simulink model "Comparativa_dinamica_ampliado_complejo"  (Simulink 8.3)
settings: Solver=ode45  StartTime=0.0  StopTime=10.0  RelTol=1e-3
settings Model: Creator=mvelasco  LastModifiedBy=mvelasco
settings DataIOCC: SignalLoggingSaveFormat=Dataset
settings DebuggingCC: UnderspecifiedInitializationDetection=Simplified  StateNameClashWarn=none
settings GRTTargetCC: CombineOutputUpdateFcns=on  GRTInterface=off

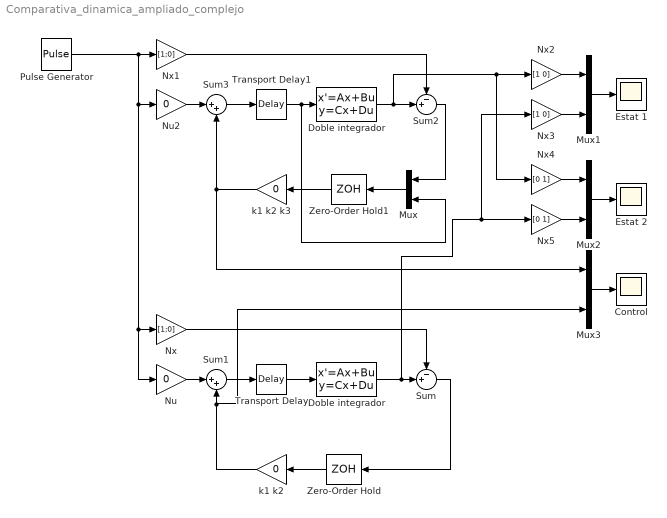
== system Comparativa_dinamica_ampliado_complejo ==
  Control : Scope
      settings: SaveName=ScopeData2
  Doble integrador : StateSpace  X0=0
  "Doble integrador " : StateSpace  X0=0
  Estat 1 : Scope
  Estat 2 : Scope
  Mux{,1..3} (4 alike) : Mux  Inputs=2
  Nu : Gain  Gain=0
  Nu2 : Gain  Gain=0
  Nx : Gain  Gain=[1;0]
  Nx1 : Gain  Gain=[1;0]
  Nx2 : Gain  Gain=[1 0]
  Nx3 : Gain  Gain=[1 0]
  Nx4 : Gain  Gain=[0 1]
  Nx5 : Gain  Gain=[0 1]
  Pulse Generator : DiscretePulseGenerator  PulseType=Time based  Amplitude=3  Period=1  PulseWidth=.5
  Sum : Sum  Inputs=-+|
  Sum1 : Sum  Inputs=|++
  Sum2 : Sum  Inputs=-+|
  Sum3 : Sum  Inputs=|++
  Transport Delay : TransportDelay
  Transport Delay1 : TransportDelay
  Zero-Order Hold : ZeroOrderHold
  Zero-Order Hold1 : ZeroOrderHold
  k1 k2 : Gain  Gain=0
  k1 k2 k3 : Gain  Gain=0
  wires:
  Pulse Generator/1 -> Nu/1, Nx/1, Nu2/1, Nx1/1
  Nx/1 -> Sum/1
  Doble integrador/1 -> Nx3/1, Nx5/1, Sum/2
  Sum/1 -> Zero-Order Hold/1
  k1 k2/1 -> Mux3/2, Sum1/2
  Nu/1 -> Sum1/1
  Sum1/1 -> Transport Delay/1
  Transport Delay/1 -> Doble integrador/1
  Zero-Order Hold/1 -> k1 k2/1
  Nx1/1 -> Sum2/1
  "Doble integrador "/1 -> Nx4/1, Nx2/1, Sum2/2
  k1 k2 k3/1 -> Mux3/1, Sum3/2
  Nu2/1 -> Sum3/1
  Sum3/1 -> Transport Delay1/1
  Transport Delay1/1 -> Mux/2, "Doble integrador "/1
  Zero-Order Hold1/1 -> k1 k2 k3/1
  Mux/1 -> Zero-Order Hold1/1
  Sum2/1 -> Mux/1
  Mux1/1 -> Estat 1/1
  Nx2/1 -> Mux1/1
  Nx3/1 -> Mux1/2
  Mux2/1 -> Estat 2/1
  Nx4/1 -> Mux2/1
  Nx5/1 -> Mux2/2
  Mux3/1 -> Control/1
